simulink library "tether002_ul"  (R2020a)
settings: Solver=VariableStepAuto  StartTime=0.0  StopTime=10.0  RelTol=1e-3
values from neighbouring files (symbols this model uses):
  initNodePos = [INITIALLINE;INITIALLINE;INITIALLINE]    [tether002_ts.m]
  initNodeVel = [zeros(1,numNodes-2);zeros(1,numNodes-2);zeros(1,numNodes-2)]    [tether002_ts.m]
  numNodes = 11    [tether002_ts.m]
undefined symbols (not defined in the file or in its folder): TotoalNodes
libraries: powerlib_meascontrol x11, nodePosToLinkPos_ul x6, dspmtrx3 x4, sharedtransform x3, simulink_extras x2
(part 4 of 4)

== matlab function tether002_ul/tether001/MATLAB Function42 ==
  data: nodePositions input; nodeForceVecs output size=[3,numNodes]; ActiveLengths input; NumberNodesActive input
function nodeForceVecs  = fcn(nodePositions, ActiveLengths, NumberNodesActive)

% clc
% clear
% nodePositions = [0,0,1,2,3,4,5,6,7,8,9;...
%            0,0,0,0,0,0,0,0,0,0,0;...
%            0,0,0,0,0,0,0,0,0,0,0];
%     
% ActiveLengths = [0,0,.01,.1,.1,.1,.1,.1,.1,.1];
% NumberNodesActive = 9;
% TotalNodes = 11;

tetherDensity = 952;
fluidDensity = 1025;
diameter = .0144;
gravity = 9.81;

% In this notation, N is the number of nodes

% Actual Length of each link 1xN-1
linkLengths = sqrt(sum(diff(nodePositions,1,2).^2));

% Number of links, scalar
numLinks = size(linkLengths,2);

% Volume of each link, 1xN-1
Volumes  = ActiveLengths.*(pi/4)*diameter^2;

% Mass of each link, 1xN-1
linkMasses = tetherDensity*Volumes;

% Net force on the links (buoyancy - gravity) on each link, 3xN-1
linkNetForceVecs = [repmat([0 0]',[1 numLinks]);(-gravity*linkMasses + gravity*fluidDensity*Volumes)];

% Net force on the nodes, 3xN
nodeForceVecs = [linkNetForceVecs(:,1) linkNetForceVecs(:,1:end-1)+linkNetForceVecs(:,2:end) linkNetForceVecs(:,end)]/2;

if linkMasses(1) == 0
    nodeForceVecs(:,1) = nodeForceVecs(:,end-NumberNodesActive+1);
    nodeForceVecs(:,end-NumberNodesActive+1) = [0;0;0];
end
% 2
% nodeForceVecs
% %BOYANCY

== matlab function tether002_ul/tether001/MATLAB Function43 ==
  data: gndNodePos input size=[3,1]; midNodePosInternal output; midNodePos input size=[3,numNodes-2]; ActiveNodes input; ActiveLengths input; airNodePos input size=[3,1]
function midNodePosInternal   = fcn(gndNodePos, midNodePos, ActiveNodes, ActiveLengths, airNodePos)

% clc
% clear
% midNodePos = [1,2,3,4,5,6,7,8,9;...
%               1,2,3.5,4,5,6,7,8,9;...
%               1,2,3,4,5,6,7,8,9];
% ActiveLengths = [1.7,1.7,1.7,1.7,1.7,1.7,1.7,1.7,1.7];
% gndNodePos = [0;0;0];
% airNodePos = [10;10;10];
% ActiveNodes = 10;

Radius = 45;

No = size(midNodePos,2)+2;
Na = ActiveNodes;

% norm(midNodePos(:,(No-Na)+2))
% if norm(midNodePos(:,(No-Na)+2))<Radius
%     Na = Na-1;
% end

% Reeled In Nodes are ground
midNodePosInternal = [gndNodePos(1)*ones(1,No-2);...
                      gndNodePos(2)*ones(1,No-2);...
                      gndNodePos(3)*ones(1,No-2)];

% Given for unalternd nodes
midNodePosInternal(:,((No-Na)+1):end) = midNodePos(:,((No-Na)+1):end);








% midlinkVecs  = diff([gndNodePos,midNodePos,airNodePos],1,2);
%  
%  
% % Find Unit Vector between given nodes
% midlinkUnitVecs = midlinkVecs./repmat(sqrt(sum((midlinkVecs.^2),1)),[3 1]);
% 
% midNodePosInternal(:,((No-Na)+1)) = gndNodePos+(ActiveLengths((No-Na)+1)*midlinkUnitVecs(:,(No-Na)+1));
% 



% nodePositions = [gndNodePos,midNodePos,airNodePos];
% linkVecs  = diff(nodePositions,1,2);
% CurrentLinkLengths = sqrt(sum(linkVecs.^2));

== matlab function tether002_ul/tether001/Subsystem1/MATLAB Function28 ==
  data: TotalForce input; Link1Forces output; OriginalLengths input; ActiveNodes input; gndNodePos input; midNodePos input; airNodePos input
function Link1Forces = fcn(TotalForce,OriginalLengths,ActiveNodes,gndNodePos,midNodePos,airNodePos)

No = length(OriginalLengths)+1;
Na = ActiveNodes;

linkVecs  = diff([gndNodePos,midNodePos,airNodePos],1,2);
  
% Find Unit Vector between given nodes
linkUnitVecs = linkVecs./repmat(sqrt(sum((linkVecs.^2),1)),[3 1]);


TopForce = TotalForce(:,(No-Na)+2)-TotalForce(:,(No-Na)+2).*linkUnitVecs(:,1);
BottomForce = TotalForce(:,(No-Na)+1);
%BottomForce = TotalForce(:,(No-Na)+2).*linkUnitVecs(:,1);



Link1Forces = [BottomForce,TopForce];



%Matching 1-2 and 2-3 Angle
% %Option 3
% r_O = [1;0;0];
% r_A = linkUnitVecs(:,1);
% 
% if ne(r_O,r_A)
%     v = cross(r_O,r_A); 
%     ssc = [0 -v(3) v(2); v(3) 0 -v(1); -v(2) v(1) 0]; 
%     A_c_O = eye(3) + ssc + ssc^2*(1-dot(r_O,r_A))/(norm(v))^2;
% else
%     A_c_O = eye(3);
% end
% 
% 
% A_c_O

== matlab function tether002_ul/tether001/Subsystem1/MATLAB Function29 ==
  data: invNodeMasses input; Link1invNodeMasses output; OriginalLengths input; ActiveNodes input
function Link1invNodeMasses = fcn(invNodeMasses,OriginalLengths,ActiveNodes)

No = length(OriginalLengths)+1;
Na = ActiveNodes;

Link1invNodeMasses = [invNodeMasses(:,1),invNodeMasses(:,(No-Na)+2)];

== matlab function tether002_ul/tether001/Subsystem1/MATLAB Function30 ==
  data: initNodeVel input; Link1initNodeVel output; OriginalLengths input; ActiveNodes input
function Link1initNodeVel = fcn(initNodeVel,OriginalLengths,ActiveNodes)

No = length(OriginalLengths)+1;
Na = ActiveNodes;

Link1initNodeVel = [initNodeVel(:,1),initNodeVel(:,(No-Na)+2)];

== matlab function tether002_ul/tether001/Subsystem1/MATLAB Function31 ==
  data: initNodePos input; Link1initNodePos output; OriginalLengths input; ActiveNodes input
function Link1initNodePos = fcn(initNodePos,OriginalLengths,ActiveNodes)

No = length(OriginalLengths)+1;
Na = ActiveNodes;

Link1initNodePos = [initNodePos(:,1),initNodePos(:,(No-Na)+2)];

== matlab function tether002_ul/tether001/Subsystem1/Hydrodynamic Force/MATLAB Function ==
  data: nodePositions input; nodeForceVecs output; nodeVelocities input; flowVel input
function nodeForceVecs = fcn(nodePositions,nodeVelocities, flowVel)
% In the notation here, N is the number of nodes, therefore you have N-1
% links between the nodes.


flowDensity = 1025;
dragCoeff = .5;
thrDiam = .0144;

% Velocity and center of links 3xN-1
linkVelocities = (nodeVelocities(:,1:end-1) + nodeVelocities(:,2:end))/2;

% Apparent flow at center of links 3xN-1
linkAppFlow = flowVel - linkVelocities; %repmat(flowVel(:),[1 size(linkVelocities,2)]) - linkVelocities;
% linkAppFlow(3,:) = 0; % Origional model zeroed z component

% Link center apparent flow magnitude 3xN-1
linkAppFlowMag = sqrt(sum(linkAppFlow.^2)); % Sum over columns

% Normalize columns to get unit vector 3xN-1
dragDirUnitVec = linkAppFlow./repmat(linkAppFlowMag,[3 1]);

% If linkAppFlowMag is zero, dragDirUnitVec will have nans, patch to fix
% that with zeros
% dragDirUnitVec(:,linkAppFlowMag==0) = zeros(3,numel(linkAppFlowMag==0));

% Dynamic pressures at link centers 1xN-1
dynPress = 0.5*flowDensity*linkAppFlowMag.^2;

% Link lengths, diff over columns 1xN-1
linkLengths = sqrt(sum(diff(nodePositions,1,2).^2));

% Unit vectors in the direction of the link 3xN-1
linkUnitVecs = diff(nodePositions,1,2)./repmat(linkLengths,[3 1]);

% Projected areas of each link
projArea = thrDiam*linkLengths.*sqrt(sum(cross(linkUnitVecs,dragDirUnitVec).^2,1));

% Drag force on links
linkForceVecs = repmat(dragCoeff*dynPress.*projArea,[3 1]).*dragDirUnitVec;

% Drag force on nodes
nodeForceVecs = [linkForceVecs(:,1) (linkForceVecs(:,1:end-1)+linkForceVecs(:,2:end)) linkForceVecs(:,end)]/2;

end

== matlab function tether002_ul/tether001/Subsystem1/MATLAB Function32 ==
  data: ReelInAcc input; Node01Vel input; OUT2 output
function OUT2 = fcn(ReelInAcc, Node01Vel)

OUT2 = -ReelInAcc*Node01Vel;

== matlab function tether002_ul/tether001/Subsystem1/MATLAB Function33 ==
  data: ReelInVel input; Node01Vel input; OUT output
function OUT = fcn(ReelInVel, Node01Vel)


OUT = -2*ReelInVel*Node01Vel;

== matlab function tether002_ul/tether001/MATLAB Function45 ==
  data: OriginalLengths input; L output; ActiveNodes input; ActiveLengths input
function L = fcn(OriginalLengths, ActiveNodes, ActiveLengths)

No = length(OriginalLengths)+1;
Na = ActiveNodes;

L = ActiveLengths((No-Na)+1);

%Streched = norm(r_BA);
% 
% if Streched>0
%     L = ActiveLengths((No-Na)+1)+(Streched-ActiveLengths((No-Na)+2))*(ActiveLengths((No-Na)+1))/Streched;
% elseif time ==0
%     L = ActiveLengths((No-Na)+1);
% else
%     L = ActiveLengths((No-Na)+1);
% end
% 
% 
% if L<0
%     L = ActiveLengths((No-Na)+1);
% end

== matlab function tether002_ul/tether001/Subsystem1/MATLAB Function35 ==
  data: ActiveLengths input; OriginalLengths input; ActiveNodes input; invL output; L output
function [invL,L] = fcn(ActiveLengths,OriginalLengths,ActiveNodes)

No = length(OriginalLengths)+1;
Na = ActiveNodes;

L = ActiveLengths(:,(No-Na)+1);

invL = 1/L;

== matlab function tether002_ul/tether001/MATLAB Function ==
  data: AccTotal input; o_a_AO_O input; ActiveNodes input; Acc output
function Acc = fcn(AccTotal,o_a_AO_O, ActiveNodes)

No = size(AccTotal,2)+2;
Na = ActiveNodes;

Acc = zeros(3,No-2);

Acc(:,((No-Na)+1):end) = [o_a_AO_O,AccTotal(:,(No-Na+2):end)];

== matlab function tether002_ul/tether001/MATLAB Function46 ==
  data: OriginalLengths input; Fx output; ActiveNodes input; Forces input; Fy output; Fz output; BoolVel input
function [Fx,Fy,Fz] = fcn(OriginalLengths, ActiveNodes, Forces, BoolVel)

No = length(OriginalLengths)+1;
Na = ActiveNodes;


Fx = Forces(1,(No-Na)+2);
Fy = Forces(2,(No-Na)+2);
Fz = Forces(3,(No-Na)+2);

== matlab function tether002_ul/tether001/MATLAB Function47 ==
  data: invNodeMasses input; Ma output; OriginalLengths input; ActiveNodes input
function Ma = fcn(invNodeMasses,OriginalLengths,ActiveNodes)

No = length(OriginalLengths)+1;
Na = ActiveNodes;

Ma = 1/invNodeMasses(1,1);

== matlab function tether002_ul/tether001/MATLAB Function49 ==
  data: Theta_dot input; Psi_dot input; Wxd output size=1; Wyd output size=1; Wzd output size=1; L input; Ld input; Fx input; Fy input; Fz input; Ma input; Mad input; Theta input; Psi input
function [Wxd,Wyd,Wzd] = fcn(Theta_dot, Psi_dot, L, Ld, Fx, Fy, Fz, Ma, Mad, Theta, Psi)

if L*Ma >= .1
    Lma = L*Ma;
else
    Lma = .1;
end


if L==0
    Wxd = 0;
    Wyd = 0;
    Wzd = 0;
else
    Wxd = 0;
    Wyd = -(Lma*cos(Theta)*sin(Theta)*Psi_dot^2 + ...
            Fz*cos(Theta) + ...
            Fx*cos(Psi)*sin(Theta) + ...
            Fy*sin(Psi)*sin(Theta) + ...
            L*Mad*Theta_dot + ...
            2*Ld*Ma*Theta_dot)/(Lma);
    Wzd = -(Fx*sin(Psi) - ...
            Fy*cos(Psi) + ...
            L*Mad*Psi_dot*cos(Theta) + ...
            2*Ld*Ma*Psi_dot*cos(Theta) - ...
            Lma*Psi_dot*Theta_dot*sin(Theta))/(Lma);
end


% if L==0
%     Wxd = 0;
%     Wyd = 0;
%     Wzd = 0;
% else
%     Wxd = 0;
%     Wyd = -(L*Ma*cos(Theta)*sin(Theta)*Psi_dot^2 + ...
%             Fz*cos(Theta) + ...
%             Fx*cos(Psi)*sin(Theta) + ...
%             Fy*sin(Psi)*sin(Theta) + ...
%             L*Mad*Theta_dot + ...
%             2*Ld*Ma*Theta_dot)/(L*Ma);
%     Wzd = -(Fx*sin(Psi) - ...
%             Fy*cos(Psi) + ...
%             L*Mad*Psi_dot*cos(Theta) + ...
%             2*Ld*Ma*Psi_dot*cos(Theta) - ...
%             L*Ma*Psi_dot*Theta_dot*sin(Theta))/(L*Ma);
% end

















% if abs(Wyd)>=10000
%     Wyd = sign(Wyd)*10000;
% end
% if abs(Wxd)>=10000
%     Wxd = sign(Wyd)*10000;
% end
% if abs(Wzd)>=10000
%     Wzd = sign(Wyd)*10000;
% end

% if isnan(Wyd)
%     Wyd = 0;
% end
% if isnan(Wxd) 
%     Wxd = 0;
% end
% if isnan(Wzd)
%     Wzd = 0;
% end

== matlab function tether002_ul/tether001/MATLAB Function23 ==
  data: Wy input; Theta_dot output; Psi_dot output; Wz input; Theta input; L input
function [Theta_dot,Psi_dot] = fcn(Wy, Wz, Theta, L)

if L==0
    Theta_dot = 0;
    Psi_dot = 0;
else
    Theta_dot = Wy;
    Psi_dot = (1/cos(Theta))*Wz;
end

== matlab function tether002_ul/tether001/Subsystem1/Weigh//Boyancy/MATLAB Function ==
  data: nodePositions input; nodeForceVecs output; unstretchedLength input
function nodeForceVecs  = fcn(nodePositions,unstretchedLength)

tetherDensity = 952;
fluidDensity = 1025;
diameter = .0144;
gravity = -9.81;

% In this notation, N is the number of nodes

% Length of each link 1xN-1
linkLengths = sqrt(sum(diff(nodePositions,1,2).^2));

% Total length of all links, assuming they're straight lines, scalar
numericalTotalLength = sum(linkLengths);

% Number of links, scalar
numLinks = size(linkLengths,2);

% Total volume based on unspooled length, scalar
analyticalTotalVol  = unstretchedLength*(pi/4)*diameter^2;

% Total mass, based on unspooled length, scalar
analyticalTotalMass = tetherDensity*analyticalTotalVol;

% Mass of each link, 1xN-1
linkMasses  = analyticalTotalMass*(linkLengths./numericalTotalLength);

% Volume of each link, 1xN-1
linkVolumes = analyticalTotalVol*(linkLengths./numericalTotalLength);

% Net force on the links (buoyancy - gravity) on each link, 3xN-1
linkNetForceVecs = [repmat([0 0]',[1 numLinks]);(-gravity*linkMasses + gravity*fluidDensity*linkVolumes)];

% Net force on the nodes, 3xN
nodeForceVecs = [linkNetForceVecs(:,1) linkNetForceVecs(:,1:end-1)+linkNetForceVecs(:,2:end) linkNetForceVecs(:,end)]/2;


end

== matlab function tether002_ul/tether001/MATLAB Function38 ==
  data: A_c_O output; Theta input; Psi input
function A_c_O = fcn(Theta, Psi)



A_c_O = [cos(Psi)*cos(Theta) ,cos(Theta)*sin(Psi) ,-sin(Theta) ;...
         -sin(Psi)           ,cos(Psi)            ,0           ;...
         cos(Psi)*sin(Theta) ,sin(Psi)*sin(Theta) ,cos(Theta)  ];

== matlab function tether002_ul/tether001/MATLAB Function44 ==
  data: o_a_AO_O output; A_c_O input; Wx input; Wxd input; Wy input; Wyd input; Wz input; Wzd input; L input; Ld input; Ldd input
function o_a_AO_O  = fcn(A_c_O, Wx, Wxd, Wy, Wyd, Wz, Wzd, L, Ld, Ldd)

O_c_A = transpose(A_c_O);

if L==0
    o_a_AO_O = [0;0;0];
else
    o_a_AO_A = [Ldd-L*(Wy^2+Wz^2)     ;...
                Wzd*L+2*Wz*Ld+Wx*Wy*L ;...
                -Wyd*L-2*Wy*Ld+Wx*Wz*L];

    o_a_AO_O = O_c_A*o_a_AO_A;
end

== matlab function tether002_ul/tether001/MATLAB Function48 ==
  data: PosTotal input; midNodePos output; VelTotal input; midNodeVel output; OriginalLengths input; ActiveNodes input; r_AO_O input; o_v_AO_O input; gndNodePos input; gndNodeVel input
function [midNodePos,midNodeVel] = fcn(PosTotal, VelTotal, OriginalLengths, ActiveNodes, r_AO_O, o_v_AO_O, gndNodePos, gndNodeVel)

No = length(OriginalLengths)+1;
Na = ActiveNodes;

midNodePos = [gndNodePos(1).*ones(1,No-2);...
              gndNodePos(2).*ones(1,No-2);...
              gndNodePos(3).*ones(1,No-2)];
midNodeVel = [gndNodeVel(1).*ones(1,No-2);...
              gndNodeVel(2).*ones(1,No-2);...
              gndNodeVel(3).*ones(1,No-2)];

if Na>2
    midNodePos(:,((No-Na)+1):end) = [r_AO_O,PosTotal(:,((No-Na)+2):end)];
    midNodeVel(:,((No-Na)+1):end) = [o_v_AO_O,VelTotal(:,((No-Na)+2):end)];
end

== matlab function tether002_ul/tether001/MATLAB Function50 ==
  data: A_c_O input; r_AO_O output; L input; time input; Air_c_O_CurrentNode input
function r_AO_O = fcn(A_c_O, L, time, Air_c_O_CurrentNode)


O_c_A = transpose(A_c_O);

if L==0
    r_AO_O = [0;0;0];
elseif time==0
	r_AO_A   = [L;...
                0;...
                0];

    r_AO_O   = Air_c_O_CurrentNode*r_AO_A;
else
    r_AO_A   = [L;...
                0;...
                0];

    r_AO_O   = O_c_A*r_AO_A;
end

== matlab function tether002_ul/tether001/MATLAB Function51 ==
  data: o_v_AO_O output; A_c_O input; Wx input; Wy input; Wz input; L input; Ld input
function o_v_AO_O  = fcn(A_c_O, Wx, Wy, Wz, L, Ld)

O_c_A = transpose(A_c_O);

if L==0
    o_v_AO_O = [0;0;0];
else
    o_v_AO_A = [Ld   ;...
                Wz*L ;...
                -Wy*L];

    o_v_AO_O = O_c_A*o_v_AO_A;
end

== matlab function tether002_ul/tether001/Velocity Reset1 ==
  data: Current input; Previous input; Bool output; Vo output; gndNodeVel input; ActiveLengths input

function [Bool,Vo]  = fcn(Current, Previous, gndNodeVel, ActiveLengths)

if Current == Previous
    Bool = -1;
else
    Bool = 1;
end

Vo = [gndNodeVel(1)*ones(1,length(ActiveLengths)-1),0;...
      gndNodeVel(2)*ones(1,length(ActiveLengths)-1),0;...
      gndNodeVel(3)*ones(1,length(ActiveLengths)-1),0];

== matlab function tether002_ul/tether001/Subsystem1/Inv Mass Matrix/MATLAB Function ==
  data: nodePositions input; invNodeMasses output; unstretchedLength input
function invNodeMasses  = fcn(nodePositions,unstretchedLength)

tetherDensity = 952;
diameter = .0144;

% In this notation, N is the number of nodes

% Length of each link 1xN-1
linkLengths = sqrt(sum(diff(nodePositions,1,2).^2));

% Total length of all links, assuming they're straight lines, scalar
numericalTotalLength = sum(linkLengths);

% Total volume based on unspooled length, scalar
analyticalTotalVol  = unstretchedLength*(pi/4)*diameter^2;

% Total mass, based on unspooled length, scalar
analyticalTotalMass = tetherDensity*analyticalTotalVol;

% Mass of each link, 1xN-1
linkMasses  = analyticalTotalMass*(linkLengths./numericalTotalLength);

% 1/mass for each node, 3xN (repmat so that we can multiply with force
% vectors concatenated into matrix later
invNodeMasses    = repmat(1./([linkMasses(1) linkMasses(1:end-1)+linkMasses(2:end) linkMasses(end)]/2),[3 1]);

end

== matlab function tether002_ul/tether001/MATLAB Function7 ==
  data: Out input; Test output; Test input
function Test = fcn(Out,Test)

Out;
Test;

== matlab function tether002_ul/tether001/MATLAB Function52 ==
  data: W_Prev input; Bool input; Vo input; ActiveLengths input; initNodeVel input; Vo output; VelocityPrevious input; ActiveNodes input; OriginalLengths input; time input; Ld input; o_v_AOPrev input
function Vo  = fcn(W_Prev, Bool, Vo, ActiveLengths,initNodeVel,VelocityPrevious, ActiveNodes, OriginalLengths, time, Ld, o_v_AOPrev)

Na = ActiveNodes;
No = length(OriginalLengths)+1;

VoNew = Vo;

Previous_VelOut = Vo(:,1:end-1);
Previous_VelOut(1:3,(No-Na)+1:(end)) = VelocityPrevious(1:3,(No-Na)+1:(end-1));
    
Previous_VelIn = Vo(:,1:end-1);

if Na > 3
    Previous_VelIn(1:3,(No-Na)+2) = o_v_AOPrev;
    Previous_VelIn(1:3,(No-Na)+3:(end)) = VelocityPrevious(1:3,(No-Na)+3:(end-1));
end

W_Prev_Sized = [W_Prev(1);W_Prev(2);W_Prev(3)];


%if all(ActiveLengths)||time==0
if time==0
    VoNew = initNodeVel;
elseif Ld<=0
    %VoNew(1:3,(No-Na)+1:end) = VelocityPrevious(1:3,(No-Na)+1:end);
    VoNew = [Previous_VelOut,W_Prev_Sized];
elseif Ld>0
    VoNew = [Previous_VelIn,[0;0;0]];
end

Vo = VoNew;


if Bool == 1
    Vo;
end

== matlab function tether002_ul/tether001/MATLAB Function53 ==
  data: O_c_A_CurrentNode output; gndNodePos input; O_c_B_NextNode output; midNodePos input; ActiveNodes input; airNodePos input; r_AO output; r_BA output
function [O_c_A_CurrentNode, O_c_B_NextNode,r_AO,r_BA] = fcn(gndNodePos, midNodePos, ActiveNodes, airNodePos)

No = size(midNodePos,2)+2;
Na = ActiveNodes;

% Reeled In Nodes are ground
midNodePosInternal = [gndNodePos(1)*ones(1,No-2);...
                      gndNodePos(2)*ones(1,No-2);...
                      gndNodePos(3)*ones(1,No-2)];

% Given for unalternd nodes
midNodePosInternal(:,((No-Na)+1):end) = midNodePos(:,((No-Na)+1):end);

% Find Vector between given nodes
midlinkVecs  = diff([gndNodePos,midNodePosInternal,airNodePos],1,2);

if Na>2
    r_AO = midlinkVecs(:,(No-Na)+1);
    r_BA = midlinkVecs(:,(No-Na)+2);
    r_BO = r_BA+r_AO;

    % Find Unit Vector between first two nodes and O and node 2
    r_AO_UNIT = r_AO./repmat(sqrt(sum((r_AO.^2),1)),[3 1]);
    r_BA_UNIT = r_BA./repmat(sqrt(sum((r_BA.^2),1)),[3 1]);
    r_BO_UNIT = r_BO./repmat(sqrt(sum((r_BO.^2),1)),[3 1]);
else
    r_AO = midlinkVecs(:,(No-Na)+1);
    r_BA = [0;0;0];
    r_BO = r_BA+r_AO;

    % Find Unit Vector between first two nodes and O and node 2
    r_AO_UNIT = r_AO./repmat(sqrt(sum((r_AO.^2),1)),[3 1]);
    r_BA_UNIT = [0;0;0];
    r_BO_UNIT = r_BO./repmat(sqrt(sum((r_BO.^2),1)),[3 1]);
end

r_O = [1;0;0];

if ne(r_O,r_BO_UNIT)
    v = cross(r_O,r_BO_UNIT); 
    ssc = [0 -v(3) v(2); v(3) 0 -v(1); -v(2) v(1) 0]; 
    B_c_O_NextNode = eye(3) + ssc + ssc^2*(1-dot(r_O,r_BO_UNIT))/(norm(v))^2;
else
    B_c_O_NextNode = eye(3);
end
O_c_B_NextNode = transpose(B_c_O_NextNode);

if ne(r_O,r_AO_UNIT)
    v = cross(r_O,r_AO_UNIT); 
    ssc = [0 -v(3) v(2); v(3) 0 -v(1); -v(2) v(1) 0]; 
    A_c_O_CurrentNode = eye(3) + ssc + ssc^2*(1-dot(r_O,r_AO_UNIT))/(norm(v))^2;
else
    A_c_O_CurrentNode = eye(3);
end
O_c_A_CurrentNode = transpose(A_c_O_CurrentNode);

== matlab function tether002_ul/tether001/Position Reset1 ==
  data: r_AOPrev input; anglesNext input; anglesPrev input; CurStepNumNodes input; Bool output; PrevStepNumNodes input; GivenInit_Pos_Angle input; Init_Pos_Angle output size=[3,numNodes-1]; Previous_Pos_Angle input; ActiveLengths input; gndNodePos input; ActiveNodes input; OriginalLengths input; time input; Ld input
function [Bool,Init_Pos_Angle] = fcn(r_AOPrev, anglesNext, anglesPrev, CurStepNumNodes, PrevStepNumNodes, GivenInit_Pos_Angle, Previous_Pos_Angle, ActiveLengths, gndNodePos, ActiveNodes, OriginalLengths, time, Ld)

Na = ActiveNodes;
No = length(OriginalLengths)+1;

if PrevStepNumNodes==0
    Nc = CurStepNumNodes;
    Np = Nc;
else
    Np = PrevStepNumNodes;
    Nc = CurStepNumNodes;
end
    
% Checks If The Current Number of Nodes Equals Previous Number of Nodes
% If not equal then reset initial conditions
if Nc == Np
    Bool = -1;
else
    Bool = 1;
end

Previous_PosOUT = [gndNodePos(1)*ones(1,length(ActiveLengths)-1);...
                   gndNodePos(2)*ones(1,length(ActiveLengths)-1);...
                   gndNodePos(3)*ones(1,length(ActiveLengths)-1)];
               
Previous_PosIN = [gndNodePos(1)*ones(1,length(ActiveLengths)-1);...
                  gndNodePos(2)*ones(1,length(ActiveLengths)-1);...
                  gndNodePos(3)*ones(1,length(ActiveLengths)-1)];

Previous_PosOUT(1:3,(No-Na)+1:end) = Previous_Pos_Angle(1:3,(No-Na)+1:(end-1));

if Na > 3
    Previous_PosIN(1:3,(No-Na)+2) = r_AOPrev;
    Previous_PosIN(1:3,(No-Na)+3:end) = Previous_Pos_Angle(1:3,(No-Na)+3:(end-1));    
end
    
Previous_AngNext = [anglesNext(2);anglesNext(1);0];
Previous_AngPrev = [anglesPrev(2);anglesPrev(1);0];


%Sets Reeled in nodes to Ground Node Position and prealocate angles
% Init_Pos_Angle = [gndNodePos(1)*ones(1,length(ActiveLengths)-1),0,0;...
%                   gndNodePos(2)*ones(1,length(ActiveLengths)-1),0,0;...
%                   gndNodePos(3)*ones(1,length(ActiveLengths)-1),0,0];

Init_Pos_Angle = [gndNodePos(1)*ones(1,length(ActiveLengths)-1),0;...
                  gndNodePos(2)*ones(1,length(ActiveLengths)-1),0;...
                  gndNodePos(3)*ones(1,length(ActiveLengths)-1),0];

              
              
%if all(ActiveLengths)||time==0 %If all nodes reeled out use given Initial Conditions              
if time==0 %If all nodes reeled out use given Initial Conditions              
    Init_Pos_Angle = GivenInit_Pos_Angle;
elseif Ld<=0 %If not, use ground positions for reeled in and previous timestep for other nodes        
    %Init_Pos_Angle(1:3,(Na-No)+2:end) = Previous_Pos_Angle(1:3,(Na-No)+2:end);
    Init_Pos_Angle = [Previous_PosOUT,Previous_AngNext];
elseif Ld>0
    Init_Pos_Angle = [Previous_PosIN,Previous_AngPrev];
end

if Bool == 1
    Init_Pos_Angle;
end

== matlab function tether002_ul/tether001/MATLAB Function24 ==
  data: R input; angles output
function  angles = fcn(R)

angles = [R(1),R(2)];

== matlab function tether002_ul/tether001/MATLAB Function11 ==
  data: angles input; Xo output; Previous_Pos input
function Xo = fcn(angles, Previous_Pos)

Xo = [Previous_Pos,ones(3,1)*angles(1),ones(3,1)*angles(2)];

== matlab function tether002_ul/tether001/MATLAB Function25 ==
  data: airNodePos input; airNodeVel input; PosPrevious input; VelPrevious input; O_c_B_NextNode input; O_c_A_CurrentNode input; ActiveNodes input; ActiveLengths input; W_Prev output; o_v_AOPrev output
function [W_Prev,o_v_AOPrev] = fcn(airNodePos, airNodeVel, PosPrevious,VelPrevious,O_c_B_NextNode, O_c_A_CurrentNode, ActiveNodes, ActiveLengths)

Na = ActiveNodes;
No = length(ActiveLengths)+1;

if Na > 3
    L = norm(PosPrevious(:,(No-Na)+2))-ActiveLengths(No-Na+1);
    V_A = O_c_B_NextNode*VelPrevious(:,(No-Na)+2);
    o_v_AOPrev = O_c_A_CurrentNode*VelPrevious(:,(No-Na)+2);
else
    L = norm(airNodePos)-ActiveLengths(No-Na+1);
    V_A = O_c_B_NextNode*airNodeVel;
    o_v_AOPrev = O_c_A_CurrentNode*airNodeVel;
end

W_Prev = [0;-V_A(3)/L;V_A(2)/L];

== matlab function tether002_ul/tether001/Subsystem1/Hydrodynamic Force2/MATLAB Function ==
  data: nodePositions input; nodeForceVecs output; nodeVelocities input; linkFlowVelVecs input; NUMBEROFNODES input
function nodeForceVecs = fcn(nodePositions, nodeVelocities, linkFlowVelVecs,NUMBEROFNODES)

thrDiam = .0144;
flowDensity = 1025;
dragCoeff = .5;

% In the notation here, N is the number of nodes, therefore you have N-1
% links between the nodes.

% Velocity and center of links 3xN-1
linkVelocities = (nodeVelocities(:,1:end-1) + nodeVelocities(:,2:end))/2;

% Apparent flow at center of links 3xN-1
linkAppFlow = linkFlowVelVecs - linkVelocities; %repmat(flowVel(:),[1 size(linkVelocities,2)]) - linkVelocities;
% linkAppFlow(3,:) = 0; % Origional model zeroed z component

% Link center apparent flow magnitude 3xN-1
linkAppFlowMag = sqrt(sum(linkAppFlow.^2)); % Sum over columns

% Normalize columns to get unit vector 3xN-1
dragDirUnitVec = linkAppFlow./repmat(linkAppFlowMag,[3 1]);

% If linkAppFlowMag is zero, dragDirUnitVec will have nans, patch to fix
% that with zeros
% dragDirUnitVec(:,linkAppFlowMag==0) = zeros(3,numel(linkAppFlowMag==0));

% Dynamic pressures at link centers 1xN-1
dynPress = 0.5*flowDensity*linkAppFlowMag.^2;

% Link lengths, diff over columns 1xN-1
linkLengths = sqrt(sum(diff(nodePositions,1,2).^2));

% Unit vectors in the direction of the link 3xN-1
linkUnitVecs = diff(nodePositions,1,2)./repmat(linkLengths,[3 1]);

% Projected areas of each link
projArea = thrDiam*linkLengths.*sqrt(sum(cross(linkUnitVecs,dragDirUnitVec).^2,1));

% Drag force on links
linkForceVecs = repmat(dragCoeff*dynPress.*projArea,[3 1]).*dragDirUnitVec;

% Drag force on nodes
nodeForceVecs = [linkForceVecs(:,1) (linkForceVecs(:,1:end-1)+linkForceVecs(:,2:end)) linkForceVecs(:,end)]/2;

%nodeForceVecs = zeros(size(nodeForceVecs));
end

== matlab function tether002_ul/tether001/MATLAB Function26 ==
  data: ActiveNodes input; OriginalNodes input size=1; gndNodePos input; airNodePos input; angles input; initNodePos input; time input; Given_Pos_Angle_IC output; AngleIC output
function [Given_Pos_Angle_IC,AngleIC] = fcn(ActiveNodes,OriginalNodes,gndNodePos,airNodePos, angles, initNodePos, time)

% if time==0
    Na = ActiveNodes;
    No = OriginalNodes;

    TetherVec = [linspace(gndNodePos(1),airNodePos(1),Na);...
                 linspace(gndNodePos(2),airNodePos(2),Na);...
                 linspace(gndNodePos(3),airNodePos(3),Na)];

    PosIC = [gndNodePos(1)*ones(1,No-2);...
             gndNodePos(2)*ones(1,No-2);...
             gndNodePos(3)*ones(1,No-2)];

    % initNodePos   
    PosIC(1,((No-Na)+1):end) = linspace(TetherVec(1,2),TetherVec(1,end-1),Na-2);
    PosIC(2,((No-Na)+1):end) = linspace(TetherVec(2,2),TetherVec(2,end-1),Na-2);
    PosIC(3,((No-Na)+1):end) = linspace(TetherVec(3,2),TetherVec(3,end-1),Na-2);
    AngleIC = [angles(1);angles(2);0];
    %Given_Pos_Angle_IC = [PosIC,AngleIC];
% else
%     Given_Pos_Angle_IC = zeros(3,11-1);
% end

    Given_Pos_Angle_IC = zeros(3,11-1);

== matlab function tether002_ul/tether001/MATLAB Function1 ==
  data: gndNodePos input; O_c_A_CurrentNode output; midNodePos input; ActiveNodes input; airNodePos input; bool input; O_c_B_NextNode output; r_AO output; r_BA output
function [O_c_A_CurrentNode, O_c_B_NextNode,r_AO,r_BA] = fcn(gndNodePos, midNodePos, ActiveNodes, airNodePos, bool)

No = size(midNodePos,2)+2;
Na = ActiveNodes;

% Reeled In Nodes are ground
midNodePosInternal = [gndNodePos(1)*ones(1,No-2);...
                      gndNodePos(2)*ones(1,No-2);...
                      gndNodePos(3)*ones(1,No-2)];

% Given for unalternd nodes
midNodePosInternal(:,((No-Na)+1):end) = midNodePos(:,((No-Na)+1):end);

% Find Vector between given nodes
midlinkVecs  = diff([gndNodePos,midNodePosInternal,airNodePos],1,2);

r_AO = midlinkVecs(:,(No-Na)+1);
r_BA = midlinkVecs(:,(No-Na)+2);
r_BO = r_BA+r_AO;

% Find Unit Vector between first two nodes and O and node 2
r_AO_UNIT = r_AO./repmat(sqrt(sum((r_AO.^2),1)),[3 1]);
r_BA_UNIT = r_BA./repmat(sqrt(sum((r_BA.^2),1)),[3 1]);
r_BO_UNIT = r_BO./repmat(sqrt(sum((r_BO.^2),1)),[3 1]);

r_O = [1;0;0];

if ne(r_O,r_BO_UNIT)
    v = cross(r_O,r_BO_UNIT); 
    ssc = [0 -v(3) v(2); v(3) 0 -v(1); -v(2) v(1) 0]; 
    B_c_O_NextNode = eye(3) + ssc + ssc^2*(1-dot(r_O,r_BO_UNIT))/(norm(v))^2;
else
    B_c_O_NextNode = eye(3);
end
O_c_B_NextNode = transpose(B_c_O_NextNode);

if ne(r_O,r_AO_UNIT)
    v = cross(r_O,r_AO_UNIT); 
    ssc = [0 -v(3) v(2); v(3) 0 -v(1); -v(2) v(1) 0]; 
    A_c_O_CurrentNode = eye(3) + ssc + ssc^2*(1-dot(r_O,r_AO_UNIT))/(norm(v))^2;
else
    A_c_O_CurrentNode = eye(3);
end
O_c_A_CurrentNode = transpose(A_c_O_CurrentNode);

== matlab function tether002_ul/tether001/MATLAB Function34 ==
  data: u input; y output
function y = fcn(u)

y = u;

== matlab function tether002_ul/tether001/MATLAB Function36 ==
  data: R input; angles output
function  angles = fcn(R)

angles = [R(1),R(2)];

== matlab function tether002_ul/tether001/MATLAB Function37 ==
  data: Mad input; node1NetFVec output size=[3,1]; o_v_AO_O input size=[3,1]; Ma input; o_a_AO_O input size=[3,1]; Fx input size=1; Fy input size=1; Fz input size=1; nodeNNetFVec output size=[3,1]; Forces input; ActiveNodes input size=1
function [node1NetFVec, nodeNNetFVec] = fcn(Mad, o_v_AO_O, Ma, o_a_AO_O, Fx, Fy, Fz, Forces, ActiveNodes)

Na = ActiveNodes;

%node1NetFVec = (Ma*o_a_AO_O+Mad*o_v_AO_O+[Fx;Fy;Fz]);
%node1NetFVec = -Ma*o_a_AO_O-Mad*o_v_AO_O+[Fx;Fy;Fz]+Forces(:,1);
%node1NetFVec = +[Fx;Fy;Fz]+Forces(:,1);
%node1NetFVec = Forces(:,1);


if Na==2
    node1NetFVec = Forces(:,1)-Ma*o_a_AO_O-Mad*o_v_AO_O;
else
    node1NetFVec = +[Fx;Fy;Fz]+Forces(:,1)-Ma*o_a_AO_O-Mad*o_v_AO_O;
end

%Ma*o_a_AO_O+Mad*o_v_AO_O

nodeNNetFVec = Forces(:,end);
%nodeNNetFVec = [-nodeNNetFVec(1);nodeNNetFVec(2);nodeNNetFVec(3)];

== matlab function tether002_ul/tether001/Subsystem1/HowManyActive4 ==
  data: OriginalLengths input; ActiveNodes output; ReeledOutLength input; ActiveLengths output; TetherLength input; OriginalNodes output
function [ActiveNodes, ActiveLengths, OriginalNodes] = fcn(OriginalLengths, ReeledOutLength, TetherLength)

OriginalNodes = length(OriginalLengths)+1;
No = OriginalNodes;

ActiveLengths = zeros(size(OriginalLengths));
L = zeros(size(ActiveLengths));
flag = false;
a = 1;

if ReeledOutLength == TetherLength
    a = a+1;
    L(1:end) = OriginalLengths(1:end);
else
    while flag == false
        if ReeledOutLength == sum(OriginalLengths(a:end))
            flag = true;
        elseif ReeledOutLength > sum(OriginalLengths(a:end))
            flag = true;
        else
            a=a+1;
        end
    end

L((a-1):end) = (ReeledOutLength/(No-a+1))*ones(1,(No-a+1));

end

ActiveNodes = nnz(L)+1;
ActiveLengths = L;

== matlab function tether002_ul/tether001/Triggered Subsystem/MATLAB Function2 ==
  data: time input; r_BA input; Lcorrected output
function Lcorrected = fcn(time, r_BA)


if time == 0
    Lcorrected = 10;
else
    Lcorrected = norm(r_BA);
end

== matlab function tether002_ul/tether001/MATLAB Function2 ==
  data: gndNodePos input; Air_c_O_CurrentNode output; airNodePos input; time input
function Air_c_O_CurrentNode = fcn(gndNodePos, airNodePos,time)

if time==0
    r_TOTAL = airNodePos-gndNodePos;
    r__TOTAL_UNIT = r_TOTAL./repmat(sqrt(sum((r_TOTAL.^2),1)),[3 1]);
    r_O = [1;0;0];

    if ne(r_O,r__TOTAL_UNIT)
        v = cross(r_O,r__TOTAL_UNIT); 
        ssc = [0 -v(3) v(2); v(3) 0 -v(1); -v(2) v(1) 0]; 
        Air_c_O_CurrentNode = eye(3) + ssc + ssc^2*(1-dot(r_O,r__TOTAL_UNIT))/(norm(v))^2;
    else
        Air_c_O_CurrentNode = eye(3);
    end
else
    Air_c_O_CurrentNode = zeros(3,3);
end


end

== matlab function tether002_ul/tether001/MATLAB Function3 ==
  data: time input; Bool input size=1; BoolOut output size=1
function BoolOut = fcn(time, Bool)

if time==0 
    BoolOut = 1;
else
    BoolOut = Bool;
end

== matlab function tether002_ul/tether001/Subsystem1/HowManyActive ==
  data: OriginalLengths input; ActiveNodes output; ReeledOutLength input; ActiveLengths output; TetherLength input
function [ActiveNodes, ActiveLengths] = fcn(OriginalLengths, ReeledOutLength, TetherLength)

% clc
% clear
% N = 11;
% TetherLength = 100;
% OriginalLengths = (100/(N-1))*ones(1,N-1);
% ReeledOutLength = 61;
% mid = [10,20,30,40,50,60,70,80,90;zeros(1,9);zeros(1,9)];

ActiveLengths = zeros(size(OriginalLengths));
L = zeros(size(ActiveLengths));
flag = false;
a = 1;
if ReeledOutLength == TetherLength
    L(1:end) = OriginalLengths(1:end);
else
    while flag == false
        if ReeledOutLength == sum(OriginalLengths(a:end))
            flag = true;
        elseif ReeledOutLength > sum(OriginalLengths(a:end))
            flag = true;
        else
            a=a+1;
        end
    end
L(1:end) = [zeros(1,a-2),OriginalLengths(a-1)-(sum(OriginalLengths((a-1):end))-ReeledOutLength),OriginalLengths(a:end)];
end

ActiveNodes = nnz(L)+1;
ActiveLengths = L;



% multi = 1000;
% 
% ReeledOutLength = round(ReeledOutLength*multi)/multi;
% 
% ActiveLengths = zeros(size(OriginalLengths));
% L = zeros(size(ActiveLengths));
% flag = false;
% a = 1;
% 
% if ReeledOutLength == TetherLength
%     L(1:end) = OriginalLengths(1:end);
% else
%     while flag == false
%     sumOrgLengths = round(sum(OriginalLengths(a:end))*multi)/multi;    
%         if ReeledOutLength==sumOrgLengths
%             flag = true;
%         elseif ReeledOutLength>sumOrgLengths
%             flag = true;
%         else
%             a=a+1;
%         end
%     end
% sumOrgLengthsm1 = round(sum(OriginalLengths((a-1):end))*multi)/multi;    
% L(1:end) = [zeros(1,a-2),OriginalLengths(a-1)-(sumOrgLengthsm1-ReeledOutLength),OriginalLengths(a:end)];
% end
% 
% % ReeledOutLength
% % ActiveNodesPrev
% ActiveNodes = nnz(L)+1;
% ActiveLengths = L;



% 
%[N-ActiveNodes,1,ActiveNodes-2]
%sum([N-ActiveNodes,1,N-(N-ActiveNodes+2)])

% [N-ActiveNodes+1,ActiveNodes-2,1]
% sum([N-ActiveNodes+1,ActiveNodes-2,1])

% [N-ActiveNodes,ActiveNodes-2]
% sum([N-ActiveNodes,ActiveNodes-2])


% [zeros(3,N-ActiveNodes),mid(:,(end-(ActiveNodes-3)):end)]

== matlab function tether002_ul/tether001/MATLAB Function4 ==
  data: R input; angles output
function  angles = fcn(R)

angles = [R(1),R(2)];

== matlab function tether002_ul/tether001/MATLAB Function5 ==
  data: angles input size=[1,2]; initNodePos input size=[3,numNodes-2]; time input size=1; ActiveNodes input size=1; OriginalNodes input size=1; gndNodePos input size=[3,1]; airNodePos input size=[3,1]; Given_Pos_Angle_IC output size=[3,numNodes-1]
function Given_Pos_Angle_IC = fcn(angles, initNodePos, time, ActiveNodes,OriginalNodes,gndNodePos,airNodePos)

Q = OriginalNodes;
if time==0
    Na = ActiveNodes;
    %%%%%%%%%%%%%%%%%%%%%%%%%%%%%%%%%%%%%%%%%
    No = 11;%OriginalNodes;
    %%%%%%%%%%%%%%%%%%%%%%%%%%%%%%%%%%%%%%%%%
    %11;%OriginalNodes;%11
    %size(gndNodePos,2)+2%11;%OriginalNodes;

    TetherVec = [linspace(gndNodePos(1),airNodePos(1),Na);...
                 linspace(gndNodePos(2),airNodePos(2),Na);...
                 linspace(gndNodePos(3),airNodePos(3),Na)];

    PosIC = [gndNodePos(1)*ones(1,No-2);...
             gndNodePos(2)*ones(1,No-2);...
             gndNodePos(3)*ones(1,No-2)];

    % initNodePos   
    PosIC(1,((No-Na)+1):end) = linspace(TetherVec(1,2),TetherVec(1,end-1),Na-2);
    PosIC(2,((No-Na)+1):end) = linspace(TetherVec(2,2),TetherVec(2,end-1),Na-2);
    PosIC(3,((No-Na)+1):end) = linspace(TetherVec(3,2),TetherVec(3,end-1),Na-2);
    
    AngleIC = [angles(1);angles(2);0];
    Given_Pos_Angle_IC = [PosIC,AngleIC];
else
    Given_Pos_Angle_IC = zeros(3,size(initNodePos,2)+1);
end 
    
% 
% 1
% Given_Pos_Angle_IC
    
% if time==0
%     AngleIC = [angles(1);angles(2);0];
%     Given_Pos_Angle_IC = [initNodePos,AngleIC];
% else
%     Given_Pos_Angle_IC = zeros(3,size(initNodePos,2)+1);
% end

== matlab function tether002_ul/tether001/MATLAB Function6 ==
  data: u input
function fcn(u)

% 2
u;

== matlab function tether002_ul/tether001/MATLAB Function15 ==
  data: u input; y output
function y = fcn(u)

y = u;

== matlab function tether002_ul/tether001/Subsystem1/MATLAB Function54 ==
  data: ReeledOutLength input; nodePos input; nodeForceVecs output; nodeVel input; ActiveLengths input; NumberNodesActive input
function nodeForceVecs  = fcn(ReeledOutLength, nodePos, nodeVel, ActiveLengths, NumberNodesActive)

% clc
% clear
% nodePos = [0,0,1,2,3,4,5,6,7,8,9;...
%            0,0,0,0,0,0,0,0,0,0,0;...
%            0,0,0,0,0,0,0,0,0,0,0];
% nodeVel = [1,1,1,1,0,0,0,0,0,0,0;...
%            1,1,1,1,0,0,0,0,0,0,0;...
%            1,1,1,1,0,0,0,0,0,0,0];       
% ActiveLengths = [0,0,.01,.1,.1,.1,.1,.1,.1,.1];
% NumberNodesActive = 9;
% TotalNodes = 11;

mass = .05;
zeta = .75;
diameter = .0144;
youngsMod = 5*10^10;

TotalNodes = size(nodePos,2);
No = TotalNodes;
Na = NumberNodesActive;

SpringConsts = zeros(1,No-1);
SpringConsts(:,(No-Na+1):end) = youngsMod*(pi/4)*(diameter^2)./ActiveLengths(1,(No-Na+1):end);
DampCoeffs = zeta*2*sqrt(SpringConsts.*mass);


linkVecs  = diff(nodePos,1,2);

linkLength = sqrt(sum(linkVecs.^2));

linkUnitVecs = zeros(3,TotalNodes-1);
linkUnitVecs(1:3,(No-Na+1):end) = linkVecs(1:3,(No-Na+1):end)./repmat(sqrt(sum((linkVecs(1:3,(No-Na+1):end).^2),1)),[3 1]);

linkLengthDeriv = dot(nodeVel(:,2:end)-nodeVel(:,1:end-1),linkUnitVecs);

springForces = SpringConsts.*(linkLength-ActiveLengths);
damperForces = DampCoeffs.*linkLengthDeriv;

totalLinkForceVec = repmat(springForces+damperForces,[3 1]).*linkUnitVecs;
nodeForceVecs = [totalLinkForceVec(:,1) diff(totalLinkForceVec,1,2) -totalLinkForceVec(:,end)];

if SpringConsts(1) == 0
    nodeForceVecs(:,1) = nodeForceVecs(:,No-Na+1);
    nodeForceVecs(:,No-Na+1) = [0;0;0];
end

== matlab function tether002_ul/tether001/Subsystem1/MATLAB Function55 ==
  data: gndNodeVel input; midNodeVel input; gndNodePos input; midNodePosInternal output; midNodePos input size=[3,numNodes-2]; ActiveNodes input; midNodeVelInternal output
function [midNodePosInternal,  midNodeVelInternal] = fcn(gndNodeVel,midNodeVel,gndNodePos, midNodePos, ActiveNodes)

% clc
% clear
% midNodePos = [1,2,3,4,5,6,7,8,9;...
%               1,2,3.5,4,5,6,7,8,9;...
%               1,2,3,4,5,6,7,8,9];
% ActiveLengths = [1.7,1.7,1.7,1.7,1.7,1.7,1.7,1.7,1.7];
% gndNodePos = [0;0;0];
% airNodePos = [10;10;10];
% ActiveNodes = 10;

%Radius = 15;

No = size(midNodePos,2)+2;
Na = ActiveNodes;

% if norm(midNodePos(:,(No-Na)+2))<Radius
%     Na = Na-1;
% end

% Reeled In Nodes are ground
midNodePosInternal = [gndNodePos(1)*ones(1,No-2);...
                      gndNodePos(2)*ones(1,No-2);...
                      gndNodePos(3)*ones(1,No-2)];
                  
midNodeVelInternal = [gndNodeVel(1)*ones(1,No-2);...
                      gndNodeVel(2)*ones(1,No-2);...
                      gndNodeVel(3)*ones(1,No-2)];
                  
% Given for unalternd nodes
midNodePosInternal(:,((No-Na)+1):end) = midNodePos(:,((No-Na)+1):end);

midNodeVelInternal(:,((No-Na)+1):end) = midNodeVel(:,((No-Na)+1):end);

== matlab function tether002_ul/tether001/Subsystem1/MATLAB Function56 ==
  data: invNodeMasses output; Activelength input; ActiveNodes input
function invNodeMasses  = fcn(Activelength,ActiveNodes)

tetherDensity = 952;
diameter = .0144;

Na = ActiveNodes;
No = length(Activelength)+1;

% Mass of each link, 1xN-1
linkMasses  = tetherDensity*(Activelength*(pi/4)*diameter^2);

% 1/mass for each node, 3xN (repmat so that we can multiply with force
% vectors concatenated into matrix later
invNodeMasses = zeros(3,No);
invNodeMasses(:,(No-Na+1):end) = repmat(1./([linkMasses((No-Na+1)) linkMasses((No-Na+1):end-1)+linkMasses((No-Na+2):end) linkMasses(end)]/2),[3 1]);

%Make Zero Inverse mass also equal to zero
for i = 1:size(invNodeMasses,2)
    if invNodeMasses(:,i) == Inf
        invNodeMasses(:,i) = zeros(3,1);
    end
end

if invNodeMasses(:,1) == 0
    invNodeMasses(:,1) = invNodeMasses(:,end-ActiveNodes+1);
    invNodeMasses(:,end-ActiveNodes+1) = [0;0;0];
end

== matlab function tether002_ul/tether001/Subsystem1/MATLAB Function57 ==
  data: nodePositions input size=[3,numNodes]; nodeVelocities input size=[3,numNodes]; flowVel input; NumberNodesActive input; nodeForceVecs output
function nodeForceVecs = fcn(nodePositions,nodeVelocities, flowVel, NumberNodesActive)
% In the notation here, N is the number of nodes, therefore you have N-1
% links between the nodes.

flowDensity = 1025;
dragCoeff = .5;
thrDiam = .0144;

TotalNodes = size(nodePositions,2);
No = TotalNodes;
Na = NumberNodesActive;

% Velocity and center of links 3xN-1
linkVelocities = (nodeVelocities(:,1:end-1) + nodeVelocities(:,2:end))/2;

% Apparent flow at center of links 3xN-1
linkAppFlow = flowVel - linkVelocities; %repmat(flowVel(:),[1 size(linkVelocities,2)]) - linkVelocities;
% linkAppFlow(3,:) = 0; % Origional model zeroed z component

% Link center apparent flow magnitude 3xN-1
linkAppFlowMag = sqrt(sum(linkAppFlow.^2)); % Sum over columns

% Normalize columns to get unit vector 3xN-1
dragDirUnitVec = linkAppFlow./repmat(linkAppFlowMag,[3 1]);
dragDirUnitVec(isnan(dragDirUnitVec)) = 0;

% If linkAppFlowMag is zero, dragDirUnitVec will have nans, patch to fix
% that with zeros
% dragDirUnitVec = zeros(3,numel(linkAppFlowMag==0));

% Dynamic pressures at link centers 1xN-1
dynPress = 0.5*flowDensity*linkAppFlowMag.^2;

linkVecs  = diff(nodePositions,1,2);

% Link lengths, diff over columns 1xN-1
linkLengths = sqrt(sum(diff(nodePositions,1,2).^2));

% Unit vectors in the direction of the link 3xN-1
linkUnitVecs = zeros(3,TotalNodes-1);
linkUnitVecs(1:3,(end-NumberNodesActive+2):end) = linkVecs(1:3,(end-NumberNodesActive+2):end)./repmat(sqrt(sum((linkVecs(1:3,(end-NumberNodesActive+2):end).^2),1)),[3 1]);

% Projected areas of each link
projArea = thrDiam*linkLengths.*sqrt(sum(cross(linkUnitVecs,dragDirUnitVec).^2,1));

% Drag force on links
linkForceVecs = repmat(dragCoeff*dynPress.*projArea,[3 1]).*dragDirUnitVec;

% Drag force on nodes
nodeForceVecs = zeros(3,TotalNodes);
nodeForceVecs(:,(TotalNodes-NumberNodesActive+1):end) = [linkForceVecs(:,(TotalNodes-NumberNodesActive+1)), (linkForceVecs(:,((TotalNodes-NumberNodesActive+1)):end-1)+linkForceVecs(:,((TotalNodes-NumberNodesActive+2)):end)) linkForceVecs(:,end)]/2;

if NumberNodesActive<TotalNodes
    nodeForceVecs(:,1) = nodeForceVecs(:,No-Na+1);
    nodeForceVecs(:,No-Na+1) = [0;0;0];
end

== matlab function tether002_ul/tether001/Subsystem1/MATLAB Function58 ==
  data: nodePositions input; ActiveLengths input; NumberNodesActive input; nodeForceVecs output
function nodeForceVecs = fcn(nodePositions,ActiveLengths, NumberNodesActive)

tetherDensity = 952;
fluidDensity = 1025;
diameter = .0144;
gravity = 9.81;

% In this notation, N is the number of nodes
Na = NumberNodesActive;
No = size(nodePositions,2);

% Actual Length of each link 1xN-1
linkLengths = sqrt(sum(diff(nodePositions,1,2).^2));

% Number of links, scalar
numLinks = size(linkLengths,2);

% Volume of each link, 1xN-1
Volumes  = ActiveLengths.*(pi/4)*diameter^2;

% Mass of each link, 1xN-1
linkMasses = tetherDensity*Volumes;

% Net force on the links (buoyancy - gravity) on each link, 3xN-1
linkNetForceVecs = [repmat([0 0]',[1 numLinks]);(-gravity*linkMasses + gravity*fluidDensity*Volumes)];

% Net force on the nodes, 3xN
nodeForceVecs = [linkNetForceVecs(:,1) linkNetForceVecs(:,1:end-1)+linkNetForceVecs(:,2:end) linkNetForceVecs(:,end)]/2;

if linkMasses(1) == 0
    nodeForceVecs(:,1) = nodeForceVecs(:,No-Na+1);
    nodeForceVecs(:,No-Na+1) = [0;0;0];
end

== matlab function tether002_ul/tether001/Position Reset2 ==
  data: CurStepNumNodes input; PrevStepNumNodes input; GivenInit_Pos input; Previous_Pos input; Bool output; Init_Pos output; ActiveLengths input; gndNodePos input; ActiveNodes input; OriginalLengths input; time input; Ld input; OUT1 output; OUT2 output; OUT3 output
function [Bool,Init_Pos,OUT1,OUT2,OUT3] = fcn(CurStepNumNodes, PrevStepNumNodes, GivenInit_Pos, Previous_Pos, ActiveLengths, gndNodePos, ActiveNodes, OriginalLengths, time, Ld)

Na = ActiveNodes;
No = length(OriginalLengths)+1;

if PrevStepNumNodes==0
    Nc = CurStepNumNodes;
    Np = Nc;
else
    Np = PrevStepNumNodes;
    Nc = CurStepNumNodes;
end
    
% Checks If The Current Number of Nodes Equals Previous Number of Nodes
% If not equal then reset initial conditions
if Nc == Np
    Bool = -1;
else
    Bool = 1;
end

Previous_PosOUT = [gndNodePos(1)*ones(1,No-2);...
                   gndNodePos(2)*ones(1,No-2);...
                   gndNodePos(3)*ones(1,No-2)];
               
Previous_PosOUT(1:3,(No-Na)+1:end) = Previous_Pos(1:3,(No-Na)+2:(end-1));
     
OUT1 = gndNodePos(1)*ones(1,No-2);
OUT2 = gndNodePos(2)*ones(1,No-2);
OUT3 = gndNodePos(3)*ones(1,No-2);

OUT1(1,(No-Na)+1:end) = Previous_Pos(1,(No-Na)+2:(end-1));
OUT2(1,(No-Na)+1:end) = Previous_Pos(2,(No-Na)+2:(end-1));
OUT3(1,(No-Na)+1:end) = Previous_Pos(3,(No-Na)+2:(end-1));

%if all(ActiveLengths)||time==0 %If all nodes reeled out use given Initial Conditions              
if time==0 %If all nodes reeled out use given Initial Conditions              
    Init_Pos = GivenInit_Pos;
else %If not, use ground positions for reeled in and previous timestep for other nodes        
    Init_Pos = Previous_PosOUT;
end



polyfit(1,1,1)

== matlab function tether002_ul/tether001/Subsystem1/Tension Reel In ==
  data: nodePos input; nodeForceVecs output; nodeVel input; CurrentLengths input; NumberNodesActive input; UnstrechedLengths input
function nodeForceVecs = fcn(nodePos, nodeVel, CurrentLengths, NumberNodesActive, UnstrechedLengths)

% clc
% clear
% nodePos = [0,0,0,0,5,6.1,7.2,8.5,9.6,10,11;...
%            0,0,0,0,0,0  ,0  ,0  ,0  ,0 ,0 ;...
%            0,0,0,0,0,0  ,0  ,0  ,0  ,0 ,0 ];
% CurrentLengths = [0,0,0,1,1,1,1,1,1,1]';
% UnstrechedLengths = [1,1,1,1,1,1,1,1,1,1]';
% NumberNodesActive = 9;
% TotalNodes = 11;
 
mass = .05;
zeta = .75;
diameter = .0144;
youngsMod = 5*10^10;

% Number of nodes
N = NumberNodesActive;
Norg = size(nodePos,2);
%nodeForceVecs = zeros(3,N);

SpringConsts = zeros(1,Norg-1);
DampCoeffs = zeros(1,Norg-1);

% Spring constant and damping coefficient for each link
SpringConsts((Norg-N+2):end) = youngsMod*(pi/4)*(diameter^2)./CurrentLengths((Norg-N+2):end);
SpringConsts(Norg-N+1) = youngsMod*(pi/4)*(diameter^2)./UnstrechedLengths((Norg-N+1));
%DampCoeffs = zeta*2*sqrt(SpringConsts*mass);

% Vector from one node to another
linkVecs  = diff(nodePos,1,2);

% Length of each link
linkLength = sqrt(sum(linkVecs.^2));

% Link direction unit vectors
linkUnitVecs = linkVecs./repmat(sqrt(sum(linkVecs.^2,1)),[3 1]);

for i = 1:size(linkUnitVecs,1)
    for j = 1:size(linkUnitVecs,2)
        if isnan(linkUnitVecs(i,j))
            linkUnitVecs(i,j) = 0;
        end
    end
end

% Rate of change of vector from one node to another
%linkLengthDeriv = dot(nodeVel(:,2:end)-nodeVel(:,1:end-1),linkUnitVecs);

% Magnitude of sprint force and damping force on each link
springForces = zeros(size(linkLength));
%damperForces  = zeros(size(linkLengthDeriv));

for i = 1:N-1
    if linkLength(i)>CurrentLengths(i)
        springForces(i) = SpringConsts(i)*(linkLength(i)-CurrentLengths(i));
        %damperForces(i) = DampCoeffs(i)*linkLengthDeriv(i);
    end
end
% Total force in each link
%totalLinkForceVec = repmat(springForces+damperForces,[3 1]).*linkUnitVecs;
totalLinkForceVec = repmat(springForces,[3 1]).*linkUnitVecs;


% Force on each node
nodeForceVecs = [totalLinkForceVec(:,1) diff(totalLinkForceVec,1,2) -totalLinkForceVec(:,end)];
nodeForceVecs(:,1) = nodeForceVecs(:,Norg-N+2);
nodeForceVecs(:,Norg-N+2) = [0;0;0];

nodeForceVecs
%nodeForceVecs = zeros(size(nodeForceVecs));
